simulink model "Comm_gatera_TEST_b"  (R2020a)
settings: Solver=VariableStepAuto  StartTime=0.0  StopTime=20  RelTol=1e-3
settings Model: DataDictionary=Registro_variables.sldd  Creator=Juan  LastModifiedBy=Juan

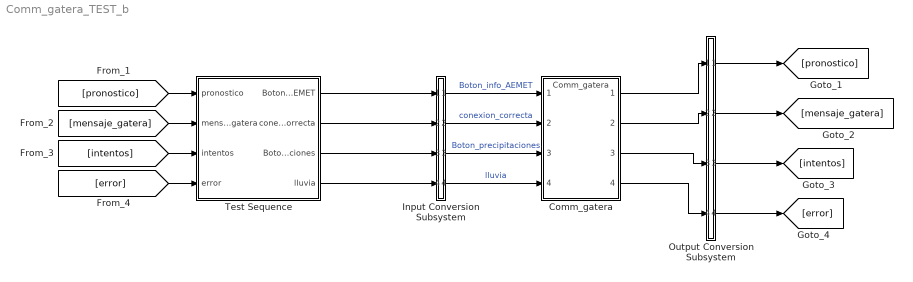
== system Comm_gatera_TEST_b ==
  Comm_gatera : ModelReference  ModelNameDialog=Comm_gatera  SimulationMode=Normal  ModelReferenceVersion=1.26
  Input Conversion Subsystem : Subsystem  Tag=__SLT_ICS__  Description=|
      | Signal spec.
      | and routing
      settings: AttributesFormatString=%<Description>
  Output Conversion Subsystem : Subsystem  Tag=__SLT_OCS__  Description=|
      | Signal spec.
      | and routing
      settings: AttributesFormatString=%<Description>
  Test Sequence : Test Sequence  TreatAsAtomicUnit=on
  wires:
  Test Sequence/1(Boton_info_AEMET) -> Input Conversion Subsystem/1(Inport_1)
  Test Sequence/2(conexion_correcta) -> Input Conversion Subsystem/2(Inport_2)
  Test Sequence/3(Boton_precipitaciones) -> Input Conversion Subsystem/3(Inport_3)
  Test Sequence/4(lluvia) -> Input Conversion Subsystem/4(Inport_4)
  [pronostico] -> Test Sequence/1(pronostico)
  [mensaje_gatera] -> Test Sequence/2(mensaje_gatera)
  [intentos] -> Test Sequence/3(intentos)
  [error] -> Test Sequence/4(error)
  Output Conversion Subsystem/1(Outport_1) -> [pronostico]
  Output Conversion Subsystem/2(Outport_2) -> [mensaje_gatera]
  Output Conversion Subsystem/3(Outport_3) -> [intentos]
  Output Conversion Subsystem/4(Outport_4) -> [error]
  Input Conversion Subsystem/1(Outport_1) -> Comm_gatera/1  "Boton_info_AEMET"
  Input Conversion Subsystem/2(Outport_2) -> Comm_gatera/2  "conexion_correcta"
  Input Conversion Subsystem/3(Outport_3) -> Comm_gatera/3  "Boton_precipitaciones"
  Input Conversion Subsystem/4(Outport_4) -> Comm_gatera/4  "lluvia"
  Comm_gatera/1 -> Output Conversion Subsystem/1(Inport_1)
  Comm_gatera/2 -> Output Conversion Subsystem/2(Inport_2)
  Comm_gatera/3 -> Output Conversion Subsystem/3(Inport_3)
  Comm_gatera/4 -> Output Conversion Subsystem/4(Inport_4)

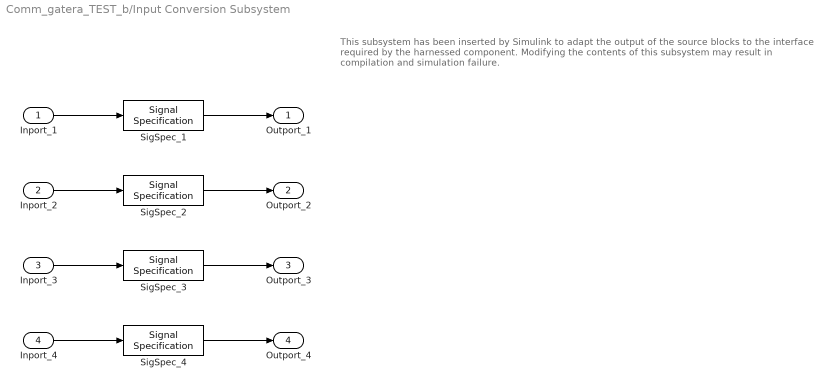
== system Comm_gatera_TEST_b/Input Conversion Subsystem ==
  note: This subsystem has been inserted by Simulink to adapt the output of the source blocks to the interface required by the harnessed component.
      |  Modifying the contents of this subsystem may result in compilation and simulation failure.
  Inport_1 : Inport
  Inport_2 : Inport  Port=2
  Inport_3 : Inport  Port=3
  Inport_4 : Inport  Port=4
  SigSpec_1 : SignalSpecification  OutDataTypeStr=boolean  Dimensions=[1]  SampleTime=[-1, 0]
  SigSpec_2 : SignalSpecification  OutDataTypeStr=boolean  Dimensions=[1]  SampleTime=[-1, 0]
  SigSpec_3 : SignalSpecification  OutDataTypeStr=boolean  Dimensions=[1]  SampleTime=[-1, 0]
  SigSpec_4 : SignalSpecification  OutDataTypeStr=double  Dimensions=[1]  SampleTime=[-1, 0]
  Outport_1 : Outport
  Outport_2 : Outport  Port=2
  Outport_3 : Outport  Port=3
  Outport_4 : Outport  Port=4
  wires:
  SigSpec_1/1 -> Outport_1/1
  Inport_1/1 -> SigSpec_1/1
  SigSpec_2/1 -> Outport_2/1
  Inport_2/1 -> SigSpec_2/1
  SigSpec_3/1 -> Outport_3/1
  Inport_3/1 -> SigSpec_3/1
  SigSpec_4/1 -> Outport_4/1
  Inport_4/1 -> SigSpec_4/1

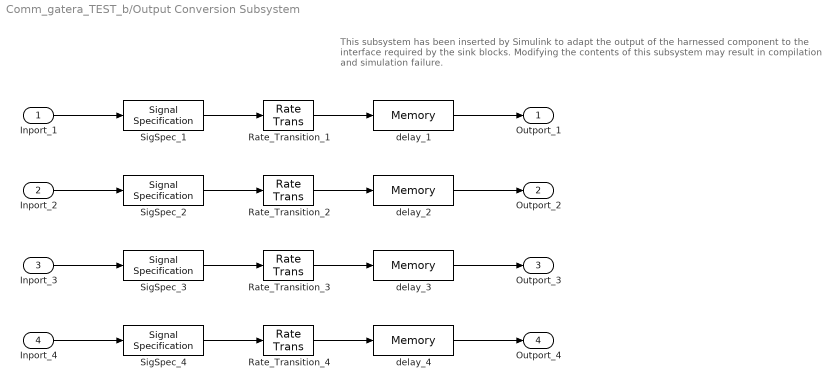
== system Comm_gatera_TEST_b/Output Conversion Subsystem ==
  note: This subsystem has been inserted by Simulink to adapt the output of the harnessed component to the interface required by the sink blocks.
      |  Modifying the contents of this subsystem may result in compilation and simulation failure.
  Inport_1 : Inport
  Inport_2 : Inport  Port=2
  Inport_3 : Inport  Port=3
  Inport_4 : Inport  Port=4
  Rate_Transition_{1..4} (4 alike) : RateTransition  OutPortSampleTimeOpt=Inherit
  SigSpec_1 : SignalSpecification  OutDataTypeStr=boolean  Dimensions=[1]
  SigSpec_2 : SignalSpecification  OutDataTypeStr=double  Dimensions=[1]
  SigSpec_3 : SignalSpecification  OutDataTypeStr=double  Dimensions=[1]
  SigSpec_4 : SignalSpecification  OutDataTypeStr=double  Dimensions=[1]
  delay_{1..4} (4 alike) : Memory
  Outport_1 : Outport
  Outport_2 : Outport  Port=2
  Outport_3 : Outport  Port=3
  Outport_4 : Outport  Port=4
  wires:
  Inport_1/1 -> SigSpec_1/1
  SigSpec_1/1 -> Rate_Transition_1/1
  Rate_Transition_1/1 -> delay_1/1
  delay_1/1 -> Outport_1/1
  Inport_2/1 -> SigSpec_2/1
  SigSpec_2/1 -> Rate_Transition_2/1
  Rate_Transition_2/1 -> delay_2/1
  delay_2/1 -> Outport_2/1
  Inport_3/1 -> SigSpec_3/1
  SigSpec_3/1 -> Rate_Transition_3/1
  Rate_Transition_3/1 -> delay_3/1
  delay_3/1 -> Outport_3/1
  Inport_4/1 -> SigSpec_4/1
  SigSpec_4/1 -> Rate_Transition_4/1
  Rate_Transition_4/1 -> delay_4/1
  delay_4/1 -> Outport_4/1

== stateflow chart Comm_gatera_TEST_b/Test Sequence ==
  settings: stateMachineType=SIMPLIFIED_MACHINE
  state Run
    %% Initialize data outputs.
    Boton_info_AEMET = false;
    conexion_correcta = false;
    Boton_precipitaciones = false;
    lluvia = 0;
  state step_1
    Boton_info_AEMET = true;
  state step_2
    conexion_correcta = true;
    Boton_precipitaciones = true;
  state step_3
    lluvia = 1;
  (default) -> Run
  Run -> step_1 : [
      | after(1,msec)
      | ]
  step_1 -> step_2 : [
      | after(2,sec)
      | ]
  step_2 -> step_3 : [
      | after(1,msec)
      | ]
  data: pronostico input boolean size=[1]; mensaje_gatera input double size=[1]; intentos input double size=[1]; error input double size=[1]; Boton_info_AEMET output boolean size=[1]; conexion_correcta output boolean size=[1]; Boton_precipitaciones output boolean size=[1]; lluvia output double size=[1]
